simulink model "sm_scissor_lift_testenv"  (R2021a)
settings: Solver=ode15s  StartTime=0.0  StopTime=50  FixedStep=5e-3  MaxStep=1e-2  RelTol=1e-3  AbsTol=1e-4  EnableMultiTasking=on
PreLoadFcn:
  | if(~exist('SCL_Par'))
  |   SCL_Par = sm_scissor_lift_param;
  | end
PostLoadFcn:
  | warning('off','mech2:compiler:topologyAnalysis:DanglingBlock');
  | warning('off','sm:sli:setup:compile:LocalSolverNotSupported');
  | warning('off','MATLAB:subscripting:noSubscriptsSpecified');
StartFcn:
  | tic;
StopFcn:
  | Elapsed_Sim_Time = toc;
  | %disp(['Elapsed Sim Time = ' num2str(Elapsed_Sim_Time')]);
values from neighbouring files (symbols this model uses):
  lift_extra_mass = 0    [startup_sm_scissor_lift.m]
undefined symbols (not defined in the file or in its folder): Local, sigbuilder_block, X, Y, Z
libraries: sm_lib x116, sm_scissor_lift_lib x29, nesl_utility x26, fl_lib x8, sh_lib x4, Contact_Forces_Lib x4, simulink x1
(part 1 of 6)
CloseFcn:
  | try,close(h1_sm_scissor_lift_testenv),end
  | clear h1_Scissor_Lift
  | try,close(h2_sm_scissor_lift_testenv),end
  | clear h2_Scissor_Lift
  | try,close(hUI_sm_scissor_lift_testenv),end
  | clear hUI_sm_scissor_lift_testenv
  | 
  | clear simlog_sm_scissor_lift_testenv
  | clear logsout_sm_scissor_lift_testenv
Description:
  | Scissor Lift Test Environment
  | 
  | Copyright 2014-2021 The MathWorks, Inc.
settings Model: Creator=smiller  LastModifiedBy=smiller
settings SolverCC: AutoScaleAbsTol=off  ConcurrentTasks=on  AlgebraicLoopSolver=TrustRegion  AutoInsertRateTranBlk=on  InsertRTBMode=Never (minimum delay)
settings DataIOCC: MaxDataPoints=10000  SaveFormat=StructureWithTime  ReturnWorkspaceOutputs=off  SignalLoggingName=logsout_sm_scissor_lift_testenv
settings OptimizationCC: BlockReduction=off  OptimizeBlockIOStorage=off  BufferReuse=off  GlobalBufferReuse=off  ExpressionFolding=off  ExpressionDepthLimit=2147483647  LocalBlockOutputs=off  OptimizeDataStoreBuffers=off  BusAssignmentInplaceUpdate=off
settings DebuggingCC: AlgebraicLoopMsg=error  UnderspecifiedInitializationDetection=Classic  MergeDetectMultiDrivingBlocksExec=none  SolverPrmCheckMsg=warning  AllowSymbolicDim=off  StateNameClashWarn=warning  PregeneratedLibrarySubsystemCodeDiagnostic=none  SFUnexpectedBacktrackingDiag=warning  SFNoUnconditionalDefaultTransitionDiag=warning  SFExecutionAtInitializationDiag=none  SFMachineParentedDataDiag=warning  ArithmeticOperatorsInVariantConditions=warning
settings ModelReferenceCC: PropagateSignalLabelsOutOfModel=off
settings SFSimCC: SimUseLocalCustomCode=off  CustomCodeUndefinedFunction=UseInterfaceOnly
settings RTWCC: Description=Generic Real-Time Target  RTWUseLocalCustomCode=off  RTWCompilerOptimization=on
settings CodeAppCC: StateflowObjectComments=on
settings GRTTargetCC: TargetLangStandard=C89/C90 (ANSI)
settings ConfigComp: CovMetricSettings=dw  CovSaveCumulativeToWorkspaceVar=on  CovSaveSingleToWorkspaceVar=on  CovExternalEMLEnable=off  CovSFcnEnable=off
settings SimscapeCC: SimscapeNormalizeSystem=off  SimscapeLogType=all  SimscapeLogSimulationStatistics=on  SimscapeLogName=simlog_sm_scissor_lift_testenv  SimscapeLogDataHistory=10000
settings ConfigurationSet: Description=SimMechanics 2G
settings DiagnosticsConfigSet: SimMechanicsUnconnectedFramePorts=none  SimMechanicsRigidlyBoundBlock=none
settings ExplorerConfigSet: InternalSimMechanicsExplorerSettings="<ExplorerConfiguration><canonicalview>default</canonicalview><AnimationSetting><BasePlaybackSpeed>1.0</BasePlaybackSpeed><PlaybackSpeedFactor>4.0</PlaybackSpeedFactor></AnimationSetting><TilePanel><TileInfo><Tiles Columns=\"2\" Count=\"3\" Rows=\"2\"><Column Left=\"2\" Weight=\"0.5\"/><Column Left=\"319\" Weight=\"0.5\"/><Column Left=\"636\"/><Row Top=\"2\" Weight=\"0.434\"/><Row Top=\"317\" Weight=\"0.566\"/><Row Top=\"726\"/><Tile Height=\"1\" Width=\"2\" X=\"0\" Y=\"0\"/><Tile Height=\"1\" Width=\"1\" X=\"0\" Y=\"1\"/><Tile Height=\"1\" Width=\"1\" X=\"1\" Y=\"1\"/></Tiles></TileInfo><SceneInfo><SceneViewer><BGColor><R>1</R><G>1</G><B>1</B></BGColor><Camera><DoPerspective>on</DoPerspective><Position><X>0.78465604483800933</X><Y>0.74998508124070185</Y><Z>5.7969918564344418</Z></Position><Center><X>1.7378942726283986</X><Y>1.0522050029517593</Y><Z>5.7969918564344409</Z></Center><Up><X>4.5985052243862679e-16</X><Y>5.259771773997932e-16</Y><Z>1</Z></Up><ViewLimDist>1</ViewLimDist><YLim>0.46630765815499858</YLim><XLim>0.95242577237540549</XLim></Camera></SceneViewer><SceneViewer><BGColor><R>1</R><G>1</G><B>1</B></BGColor><Camera><DoPerspective>off</DoPerspective><Position><X>0.019999865036961495</X><Y>-3.7807005970336149e-08</Y><Z>11.13211424643969</Z></Position><Center><X>0.019999865036961495</X><Y>-3.7807005970336149e-08</Y><Z>3.4806946063285658</Z></Center><Up><X>0</X><Y>1</Y><Z>-0</Z></Up><ViewLimDist>1</ViewLimDist><YLim>6.1531750545026354</YLim><XLim>4.7379447919670294</XLim></Camera></SceneViewer><SceneViewer><BGColor><R>1</R><G>1</G><B>1</B></BGColor><Camera><DoPerspective>off</DoPerspective><Position><X>1.0546030947508469</X><Y>-9.8853504412716475</Y><Z>4.0090833581699536</Z></Position><Center><X>1.0546030947508469</X><Y>-2.1392246596363407e-07</Y><Z>4.0090833581699536</Z></Center><Up><X>0</X><Y>-0</Y><Z>1</Z></Up><ViewLimDist>1</ViewLimDist><YLim>4.9840717941471349</YLim><XLim>3.8377352814932939</XLim></Camera></SceneViewer></SceneInfo></TilePanel><MechEditorPanel><Cameras><Camera><Id>Camera1</Id><Value><Name>Platform</Name><NativeCamera><PositionTrackingFeature>Scissor_Lift.Platform.Fixed.Cage.Transform_Camera.F</PositionTrackingFeature><CenterTrackingFeature>Scissor_Lift.Platform.Fixed.Cage.Transform_Camera.F</CenterTrackingFeature><UpVectorTrackingFeature>Scissor_Lift.Platform.Fixed.Cage.Transform_Camera.F</UpVectorTrackingFeature><CenterTrackingOrigin>off</CenterTrackingOrigin><CenterTrackingDirection>-Y</CenterTrackingDirection><UpVectorTrackingDirection>+Z</UpVectorTrackingDirection></NativeCamera></Value></Camera></Cameras><GfxPanelCameraMap><MapElement CameraMLId=\"Camera1\" GfxPanelIndex=\"0\"/></GfxPanelCameraMap><VideoCreator><PlaybackSpeedRatio>1.0</PlaybackSpeedRatio><FrameRate>30</FrameRate><VideoFormat>Motion JPEG AVI</VideoFormat><FrameSize>auto</FrameSize></VideoCreator></MechEditorPanel></ExplorerConfiguration>"

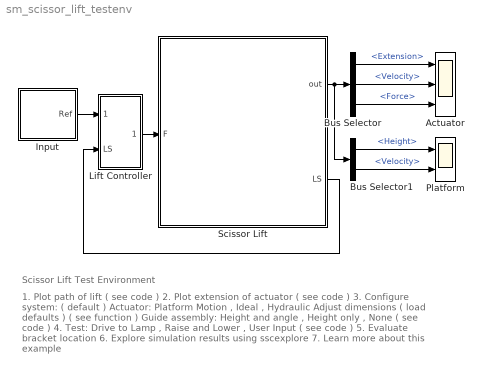
== system sm_scissor_lift_testenv ==
  note: Scissor Lift Test Environment
  note: 1. Plot path of lift ( see code )
      | 2. Plot extension of actuator ( see code )
      | 3. Configure system: ( default )
      | Actuator: Platform Motion , Ideal , Hydraulic
      | Adjust dimensions ( load defaults ) ( see function )
      | Guide assembly: Height and angle , Height only , None ( see code )
      | 4. Test: Drive to Lamp , Raise and Lower , User Input ( see code )
      | 5. Evaluate bracket location
      | 6. Explore simulation results using sscexplore
      | 7. Learn more about this example
  Actuator : Scope  NumInputPorts=3
  Bus Selector : BusSelector  OutputSignals=Actuator.Extension,Actuator.Velocity,Actuator.Force
  Bus Selector1 : BusSelector  OutputSignals=Platform.Height,Platform.Velocity
  Input : Subsystem  Variant=on  VariantControlMode=label  VariantControl=Variant1  LabelModeActiveChoice=Test_Input
      settings: AttributesFormatString=%<ActiveVariant>
      mask Display:
      | blk = find_system(gcbh, 'SearchDepth', 1, 'Parent', gcb, 'VariantObject', get_param(gcb,'activevariant'));
      | eval(get_param(blk, 'MaskDisplay'));
  Lift Controller : Subsystem
  Platform : Scope  NumInputPorts=2
  Scissor Lift : Subsystem  Tag=PublishSubsystem
      mask Display:
      | image('Scissor_Lift_3Stage_Full_IMAGE.jpg');
      | %port_label('input',1,'F');
      | %port_label('output',1,'pv');
  wires:
  Lift Controller/1(Cmd) -> Scissor Lift/1(F)
  Bus Selector/2 -> Actuator/2  "<Velocity>"
  Scissor Lift/2(LS) -> Lift Controller/2(LS)
  Input/1(" Ref") -> Lift Controller/1(Ref)
  Bus Selector/3 -> Actuator/3  "<Force>"
  Scissor Lift/1(out) -> Bus Selector1/1, Bus Selector/1
  Bus Selector1/1 -> Platform/1  "<Height>"
  Bus Selector1/2 -> Platform/2  "<Velocity>"
  Bus Selector/1 -> Actuator/1  "<Extension>"

== system sm_scissor_lift_testenv/Input ==
  Dashboard : Subsystem  VariantControl=Dashboard
      mask Display: image(imread('Scissor_Lift_Input_Dashboard_IMAGE.jpg'));
  Input : Subsystem  VariantControl=Test_Input
      mask Display: image('Scissor_Lift_Input_TestSequence_IMAGE.jpg');
  " Ref" : Outport  VectorParamsAs1DForOutWhenUnconnected=off

== system sm_scissor_lift_testenv/Lift Controller ==
  note: Copyright 2011-2021 The MathWorks, Inc.
  Ref : Inport
  LS : Inport  Port=2
  Bus Creator : BusCreator  Inputs=4
  Bus Selector : BusSelector  OutputSignals=Lift,Drive,Steer,Extend
  Bus Selector1 : BusSelector  OutputSignals=LS Height
  Full : Constant  Value=10
  Gain : Gain  Gain=0.5
  Gain1 : Gain  Gain=0.5
  Integrator : Integrator
  Integrator1 : Integrator
  Limit : Constant  Value=5
  Max Trq : Switch  Criteria=u2 > Threshold
  Product : Product
  Saturation : Saturate  UpperLimit=SCL_Par.Platform.Ext.Length*0.6/100  LowerLimit=0
  Cmd : Outport  VectorParamsAs1DForOutWhenUnconnected=off
  wires:
  Ref/1 -> Bus Selector/1
  LS/1 -> Bus Selector1/1
  Bus Selector/1 -> Bus Creator/1  "<Lift>"
  Bus Selector/2 -> Product/2  "<Drive>"
  Bus Selector/3 -> Gain/1  "<Steer>"
  Bus Creator/1 -> Cmd/1  "Cmd"
  Full/1 -> Max Trq/3
  Limit/1 -> Max Trq/1
  Max Trq/1 -> Product/1
  Product/1 -> Bus Creator/2  "Drive"
  Bus Selector1/1 -> Max Trq/2  "<LS Height>"
  Gain/1 -> Integrator/1
  Integrator/1 -> Bus Creator/3  "Steer"
  Bus Selector/4 -> Gain1/1  "<Extend>"
  Gain1/1 -> Integrator1/1
  Integrator1/1 -> Saturation/1
  Saturation/1 -> Bus Creator/4  "Extend"

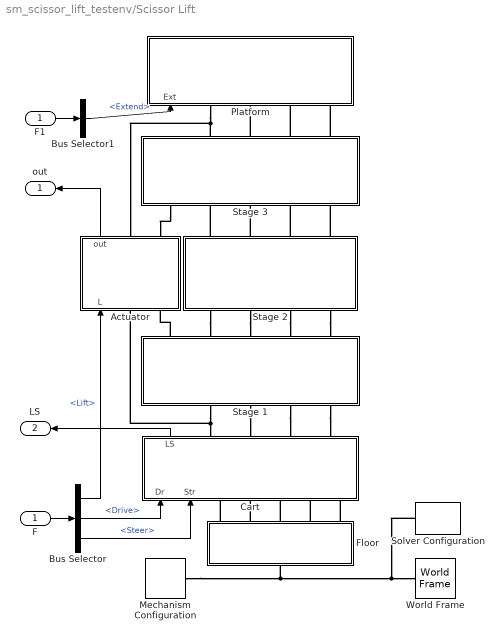
== system sm_scissor_lift_testenv/Scissor Lift ==
  F : Inport
  Actuator : Subsystem
      mask Display:
      | curblk = gcb;
      | blk = find_system([curblk '/Actuator'], 'SearchDepth', 1, 'Parent', [curblk '/Actuator'], 'VariantObject', get_param([curblk '/Actuator'],'activevariant'));
      | eval(char(get_param(blk, 'MaskDisplay')));
  Bus Selector : BusSelector  OutputSignals=Lift,Drive,Steer
  Bus Selector1 : BusSelector  OutputSignals=Extend
  Cart : Subsystem
      mask Display: image('sm_scissor_lift_cart_IMAGE.png');
  F1 : InportShadow
  Floor : Subsystem  Tag=PublishSubsystem
      mask Display: image('sm_scissor_lift_floor_IMAGE.png');
  Mechanism Configuration : sm_lib/Utilities/Mechanism Configuration  UniformGravity=Constant  GravityVector=[0 0 -9.81]  GravityVectorUnits=m/s^2  GravityUnits=m/s^2  LinearizationDelta=0.001  JointModeTransitionNonlinearIterations=2
  Platform : Subsystem
      mask Display: image('sm_scissor_lift_platform_IMAGE.png');
  Solver Configuration : nesl_utility/Solver Configuration  PhysicalDomain=network_engine_domain  SubClassName=solver  LeftPortType=input  RightPortType=generic  Tones=[]  Harmonics=[]  SimulateNoise=off  Profile=off  UseLocalSampling=off  EnableSwitchedLinearOptims=on  FrequencyDomain=off  UseCCode=off  RelTol=0.001  AbsTol=1e-06  MinStep=1e-09  ToWorkspace=off  RevertToSquareIcSolve=off  NumHomotopyIterations=100  PhasorMode=off  PhasorModeNumHarmonics=1  DoDC=off  ResidualTolerance=1e-9  UseLocalSolver=off  LocalSolverChoice=NE_BACKWARD_EULER_ADVANCER  LocalSolverSampleTime=.001  DoFixedCost=off  MaxNonlinIter=3  MaxModeIter=2  ComputeImpulses=off  ImpulseIterations=2  LinearAlgebra=Sparse  EquationFormulation=NE_TIME_EF  DelaysMemoryBudget=1024  AutomaticFiltering=on  FilteringTimeConstant=0.001  PartitionStorageMethod=AS_NEEDED  PartitionMemoryBudget=1024  PartitionMethod=FAST
      settings: SourceProductBaseCode=PW,SS
  Stage 1 : Subsystem  Tag=PublishSubsystem
      mask Display: image('sm_scissor_lift_stage1_IMAGE.png');
  Stage 2 : Subsystem
      mask Display: image('sm_scissor_lift_stage2_IMAGE.png');
  Stage 3 : Subsystem
      mask Display: image('sm_scissor_lift_stage3_IMAGE.png');
  World Frame : sm_lib/Frames and Transforms/World Frame
  out : Outport  VectorParamsAs1DForOutWhenUnconnected=off
  LS : Outport  Port=2  VectorParamsAs1DForOutWhenUnconnected=off
  wires:
  Actuator/1(out) -> out/1
  F/1 -> Bus Selector/1
  Bus Selector/1 -> Actuator/1(L)  "<Lift>"
  Bus Selector/2 -> Cart/1(Dr)  "<Drive>"
  Bus Selector/3 -> Cart/2(Str)  "<Steer>"
  Cart/1(LS) -> LS/1
  F1/1 -> Bus Selector1/1
  Bus Selector1/1 -> Platform/1(Ext)  "<Extend>"
  connections:
  Stage 1/LConn1 -- Actuator/LConn2
  Stage 3/RConn1 -- Actuator/RConn2
  Actuator/LConn1 -- Stage 1/RConn2 -- Cart/RConn1
  Stage 1/RConn3 -- Cart/RConn2
  Stage 1/RConn4 -- Cart/RConn3
  Stage 1/RConn5 -- Cart/RConn4
  Mechanism Configuration/RConn1 -- Solver Configuration/RConn1 -- World Frame/RConn1 -- Floor/RConn1
  Platform/LConn1 -- Stage 3/LConn2 -- Actuator/RConn1
  Stage 3/LConn3 -- Platform/LConn2
  Stage 3/LConn4 -- Platform/LConn3
  Stage 3/LConn5 -- Platform/LConn4
  Floor/LConn4 -- Cart/LConn4
  Floor/LConn3 -- Cart/LConn3
  Floor/LConn1 -- Cart/LConn1
  Floor/LConn2 -- Cart/LConn2
  Floor/LConn5 -- Cart/LConn5
  Stage 2/LConn4 -- Stage 3/RConn5
  Stage 2/LConn2 -- Stage 3/RConn3
  Stage 2/RConn1 -- Stage 1/LConn2
  Stage 2/RConn2 -- Stage 1/LConn3
  Stage 2/LConn1 -- Stage 3/RConn2
  Stage 2/RConn3 -- Stage 1/LConn4
  Stage 2/RConn4 -- Stage 1/LConn5
  Stage 2/LConn3 -- Stage 3/RConn4

== system sm_scissor_lift_testenv/Input/Dashboard ==
  note: Use Simulation Pacing to make the simulation in soft real-time so that you can use the manual controls below
  Bus Creator : BusCreator  Inputs=4
  Drive : Constant  Value=0
  Extend : Constant  Value=0
  Lift : Constant  Value=0
  Push Button : PushButtonBlock  ButtonText=Up
  Push Button1 : PushButtonBlock  ButtonText=Down  OnValue=-1
  Push Button2 : PushButtonBlock  ButtonText=Forward
  Push Button3 : PushButtonBlock  ButtonText=Reverse  OnValue=-1
  Push Button4 : PushButtonBlock  ButtonText=Left
  Push Button5 : PushButtonBlock  ButtonText=Right  OnValue=-1
  Push Button6 : PushButtonBlock  ButtonText=Retract  OnValue=-1
  Push Button7 : PushButtonBlock  ButtonText=Extend
  Steer : Constant  Value=0
  Ref : Outport  VectorParamsAs1DForOutWhenUnconnected=off
  wires:
  Lift/1 -> Bus Creator/1  "Lift"
  Drive/1 -> Bus Creator/2  "Drive"
  Bus Creator/1 -> Ref/1  "Ref"
  Steer/1 -> Bus Creator/3  "Steer"
  Extend/1 -> Bus Creator/4  "Extend"

== system sm_scissor_lift_testenv/Input/Input ==
  Bus Creator : BusCreator  Inputs=4
  Signal Builder : Subsystem  Tag=STV Subsys  LoadFcn=sigbuilder_block('load');  StartFcn=sigbuilder_block('start');  StopFcn=sigbuilder_block('stop');  ClipboardFcn=sigbuilder_block('clipboard');  mask(Sigbuilder block){tuvar=[0:10]}
      mask help: Simulink:masks:SigbuilderBlock_MD
      mask init:
      | if ~strcmp(get_param(bdroot(gcbh),'SimulationStatus'),'stopped') tuvar = sigbuilder_block('maskInit'); end
      settings: CopyFcn=sigbuilder_block('copy');  DeleteFcn=sigbuilder_block('delete');  ModelCloseFcn=sigbuilder_block('modelClose');  PreSaveFcn=sigbuilder_block('preSave');  PauseFcn=sigbuilder_block('pause');  ContinueFcn=sigbuilder_block('continue');  NameChangeFcn=sigbuilder_block('namechange');  OpenFcn=sigbuilder_block('open',[49.8 117.6 550.8 438.6 ]);  CloseFcn=sigbuilder_block('close');
      mask Display: plot(0, 0, 100, 100,[2, 2, 32, 32, 2], [68, 8, 8, 68, 68],[32, 2], [38, 38], [32, 19, 2],[53, 60, 44], [32, 17, 17, 2],[16, 16, 31, 31]);txt = getActiveGroup(gcbh);text(2, 100, txt,'verticalAlignment', 'top');
  Ref : Outport  VectorParamsAs1DForOutWhenUnconnected=off
  wires:
  Signal Builder/3(Steer) -> Bus Creator/3  "Steer"
  Bus Creator/1 -> Ref/1  "Ref"
  Signal Builder/2(Drive) -> Bus Creator/2  "Drive"
  Signal Builder/1(Lift) -> Bus Creator/1  "Lift"
  Signal Builder/4(Extend) -> Bus Creator/4  "Extend"

== system sm_scissor_lift_testenv/Scissor Lift/Actuator ==
  L : Inport
  Actuator : Subsystem  Variant=on  VariantControlMode=label  LabelModeActiveChoice=Ideal
      settings: AttributesFormatString=%<ActiveVariant>
      mask Display:
      | curblk = gcb;
      | 
      | parentblk = get_param(curblk,'Parent');
      | parblk_name = char(get_param(parentblk,'Name'));
      | set_param(parentblk,'Name',parblk_name);
      | 
      | 
      | blk = find_system(gcbh, 'SearchDepth', 1, 'Parent', gcb, 'VariantObject', get_param(gcb,'activevariant'));
      | eval(get_param(blk, 'MaskDisplay'));
  Cylinder Collar : sm_scissor_lift_lib/Collar  collar_length=SCL_Par.Act.Collar.Length  collar_radius=SCL_Par.Act.Collar.Radius  cylinder_length=SCL_Par.Act.Cylinder.Length  cylinder_radius=SCL_Par.Act.Cylinder.Radius  cylinder_ori=Local +Z  material_density=SCL_Par.Act.Collar.Density  material_color=SCL_Par.Act.Collar.Color  material_opacity=SCL_Par.Act.Collar.Opacity
      settings: SourceProductName=Simscape Scissor Lift Library
  Piston : Subsystem
      mask Display: image('Piston_Shaft_IMAGE.jpg');
  Piston Collar : sm_scissor_lift_lib/Collar  collar_length=SCL_Par.Act.Collar.Length  collar_radius=SCL_Par.Act.Collar.Radius  cylinder_length=SCL_Par.Act.Piston_Seat.Length  cylinder_radius=SCL_Par.Act.Piston_Seat.Radius  cylinder_ori=Local -Z  material_density=SCL_Par.Act.Collar.Density  material_color=SCL_Par.Act.Collar.Color  material_opacity=SCL_Par.Act.Collar.Opacity
      settings: SourceProductName=Simscape Scissor Lift Library
  Rev Bracket1 Cyl : sm_lib/Joints/Revolute Joint  JointMode=Normal  SenseConstraintForce=off  SenseConstraintForceX=off  SenseConstraintForceY=off  SenseConstraintForceZ=off  SenseConstraintTorque=off  SenseConstraintTorqueX=off  SenseConstraintTorqueY=off  SenseConstraintTorqueZ=off  SenseTotalForce=off  SenseTotalForceX=off  SenseTotalForceY=off  SenseTotalForceZ=off  SenseTotalTorque=off  SenseTotalTorqueX=off  SenseTotalTorqueY=off  SenseTotalTorqueZ=off  CompositeWrenchDir=FollowerOnBase  CompositeWrenchFrame=BaseFrame  EquilibriumPosition=0  EquilibriumPositionUnits=rad  SpringStiffness=0  SpringStiffnessUnits=N*m/rad  DampingCoefficient=0  DampingCoefficientUnits=N*m/(rad/s)  TorqueActuationMode=NoTorque  MotionActuationMode=ComputedMotion  SensePosition=off  SenseVelocity=off  SenseAcceleration=off  SenseTorqueForce=off  SenseLowerLimitTorqueForce=off  SenseUpperLimitTorqueForce=off  LowerLimitSpecify=off  LowerLimitBound=-90  LowerLimitBoundUnits=deg  LowerLimitStiffness=1e4  LowerLimitStiffnessUnits=N*m/deg  LowerLimitDamping=10  LowerLimitDampingUnits=N*m/(deg/s)  LowerLimitTransitionRegionWidth=0.1  LowerLimitTransitionRegionWidthUnits=deg  UpperLimitSpecify=off  UpperLimitBound=90  UpperLimitBoundUnits=deg  UpperLimitStiffness=1e4  UpperLimitStiffnessUnits=N*m/deg  UpperLimitDamping=10  UpperLimitDampingUnits=N*m/(deg/s)  UpperLimitTransitionRegionWidth=0.1  UpperLimitTransitionRegionWidthUnits=deg  PositionTargetSpecify=off  PositionTargetPriority=High  PositionTargetValue=0  PositionTargetValueUnits=rad  VelocityTargetSpecify=off  VelocityTargetPriority=High  VelocityTargetValue=0  VelocityTargetValueUnits=rad/s
  Rev Bracket2 Cyl : sm_lib/Joints/Revolute Joint  JointMode=Normal  SenseConstraintForce=off  SenseConstraintForceX=off  SenseConstraintForceY=off  SenseConstraintForceZ=off  SenseConstraintTorque=off  SenseConstraintTorqueX=off  SenseConstraintTorqueY=off  SenseConstraintTorqueZ=off  SenseTotalForce=off  SenseTotalForceX=off  SenseTotalForceY=off  SenseTotalForceZ=off  SenseTotalTorque=off  SenseTotalTorqueX=off  SenseTotalTorqueY=off  SenseTotalTorqueZ=off  CompositeWrenchDir=FollowerOnBase  CompositeWrenchFrame=BaseFrame  EquilibriumPosition=0  EquilibriumPositionUnits=rad  SpringStiffness=0  SpringStiffnessUnits=N*m/rad  DampingCoefficient=0  DampingCoefficientUnits=N*m/(rad/s)  TorqueActuationMode=NoTorque  MotionActuationMode=ComputedMotion  SensePosition=off  SenseVelocity=off  SenseAcceleration=off  SenseTorqueForce=off  SenseLowerLimitTorqueForce=off  SenseUpperLimitTorqueForce=off  LowerLimitSpecify=off  LowerLimitBound=-90  LowerLimitBoundUnits=deg  LowerLimitStiffness=1e4  LowerLimitStiffnessUnits=N*m/deg  LowerLimitDamping=10  LowerLimitDampingUnits=N*m/(deg/s)  LowerLimitTransitionRegionWidth=0.1  LowerLimitTransitionRegionWidthUnits=deg  UpperLimitSpecify=off  UpperLimitBound=90  UpperLimitBoundUnits=deg  UpperLimitStiffness=1e4  UpperLimitStiffnessUnits=N*m/deg  UpperLimitDamping=10  UpperLimitDampingUnits=N*m/(deg/s)  UpperLimitTransitionRegionWidth=0.1  UpperLimitTransitionRegionWidthUnits=deg  PositionTargetSpecify=off  PositionTargetPriority=High  PositionTargetValue=0  PositionTargetValueUnits=rad  VelocityTargetSpecify=off  VelocityTargetPriority=High  VelocityTargetValue=0  VelocityTargetValueUnits=rad/s
  Transform From Cart : sm_lib/Frames and Transforms/Rigid Transform  TranslationMethod=None  TranslationStandardOffset=0  TranslationLengthUnit=m  TranslationStandardAxis=+X  TranslationCartesianOffset=[0 0 0]  TranslationROffset=0  TranslationROffsetUnits=m  TranslationZOffset=0  TranslationZOffsetUnits=m  TranslationThetaOffset=0  TranslationThetaOffsetUnits=deg  RotationMethod=StandardAxis  RotationAngleUnits=deg  RotationStandardAxis=+X  RotationAngle=90  RotationArbitraryAxis=[0 0 1]  FollAlignAxisA=+X  BaseAlignAxisA=+Y  FollAlignAxisB=+Y  BaseAlignAxisB=+Z  RotationSequenceAxes=FollowerAxes  RotationSequence=XYX  RotationSequenceAngles=[0 0 0]  RotationSequenceAnglesUnits=deg  RotationMatrix=[1 0 0; 0 1 0; 0 0 1]
  Transform From Platform : sm_lib/Frames and Transforms/Rigid Transform  TranslationMethod=None  TranslationStandardOffset=0  TranslationLengthUnit=m  TranslationStandardAxis=+X  TranslationCartesianOffset=[0 0 0]  TranslationROffset=0  TranslationROffsetUnits=m  TranslationZOffset=0  TranslationZOffsetUnits=m  TranslationThetaOffset=0  TranslationThetaOffsetUnits=deg  RotationMethod=StandardAxis  RotationAngleUnits=deg  RotationStandardAxis=+X  RotationAngle=90  RotationArbitraryAxis=[0 0 1]  FollAlignAxisA=+X  BaseAlignAxisA=+Y  FollAlignAxisB=+Y  BaseAlignAxisB=+Z  RotationSequenceAxes=FollowerAxes  RotationSequence=XYX  RotationSequenceAngles=[0 0 0]  RotationSequenceAnglesUnits=deg  RotationMatrix=[1 0 0; 0 1 0; 0 0 1]
  C : PMIOPort  Side=Left
  P : PMIOPort  Port=2  Side=Right
  F : PMIOPort  Port=3  Side=Right
  B : PMIOPort  Port=4  Side=Left
  out : Outport  VectorParamsAs1DForOutWhenUnconnected=off
  wires:
  L/1 -> Actuator/1(L)
  Actuator/1(Out) -> out/1
  connections:
  Cylinder Collar/LConn1 -- Rev Bracket1 Cyl/RConn1
  Piston Collar/RConn1 -- Piston/LConn1
  Rev Bracket2 Cyl/RConn1 -- Piston Collar/LConn1
  F/RConn1 -- Rev Bracket2 Cyl/LConn1
  Rev Bracket1 Cyl/LConn1 -- B/RConn1
  Actuator/RConn2 -- Piston/RConn1
  Actuator/LConn2 -- Cylinder Collar/RConn1
  C/RConn1 -- Transform From Cart/LConn1
  P/RConn1 -- Transform From Platform/LConn1
  Transform From Cart/RConn1 -- Actuator/LConn1
  Transform From Platform/RConn1 -- Actuator/RConn1

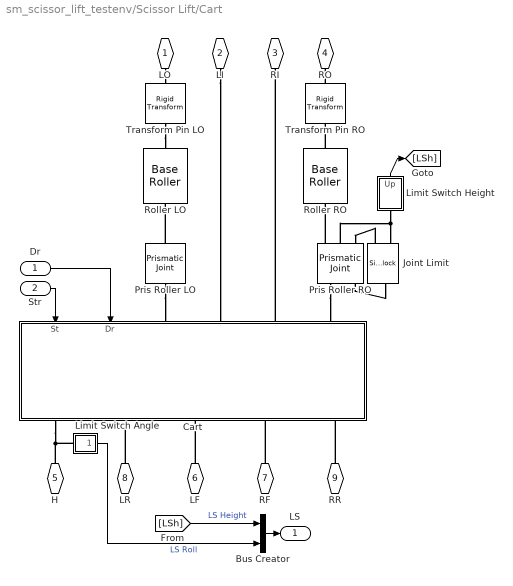
== system sm_scissor_lift_testenv/Scissor Lift/Cart ==
  Dr : Inport
  Str : Inport  Port=2
  Bus Creator : BusCreator  Inputs=2
  Cart : Subsystem
      mask Display: image('Scissor_Lift_Cart_IMAGE.jpg');
  Joint Limit : SimscapeComponentBlock  SourceFile=translational_hardstop  ComponentPath=translational_hardstop  ComponentVariants=translational_hardstop  ComponentVariantNames=translational_hardstop  ClassName=translational_hardstop  SchemaVersion=1  upper_bnd=SCL_Par.Roller.Hardstop.UB cm  lower_bnd=SCL_Par.Roller.Hardstop.LB cm  stiff_up=SCL_Par.Roller.Hardstop.Stiffness N/m  stiff_low=SCL_Par.Roller.Hardstop.Stiffness N/m  D_up=SCL_Par.Roller.Hardstop.Damping N/(m/s)  D_low=SCL_Par.Roller.Hardstop.Damping N/(m/s)
      settings: CopyFcn=simscape.engine.sli.internal.componentblockcallback(gcbh,'COPY')  PreCopyFcn=simscape.engine.sli.internal.componentblockcallback(gcbh,'PRECOPY')  PreDeleteFcn=simscape.engine.sli.internal.componentblockcallback(gcbh,'PREDELETE')
      mask Type: Translational Hard Stop
  Limit Switch Angle : Subsystem
  Limit Switch Height : Subsystem
  Pris Roller LO : sm_lib/Joints/Prismatic Joint  JointMode=Normal  SenseConstraintForce=off  SenseConstraintForceX=off  SenseConstraintForceY=off  SenseConstraintForceZ=off  SenseConstraintTorque=off  SenseConstraintTorqueX=off  SenseConstraintTorqueY=off  SenseConstraintTorqueZ=off  SenseTotalForce=off  SenseTotalForceX=off  SenseTotalForceY=off  SenseTotalForceZ=off  SenseTotalTorque=off  SenseTotalTorqueX=off  SenseTotalTorqueY=off  SenseTotalTorqueZ=off  CompositeWrenchDir=FollowerOnBase  CompositeWrenchFrame=BaseFrame  EquilibriumPosition=0  EquilibriumPositionUnits=m  SpringStiffness=0  SpringStiffnessUnits=N/m  DampingCoefficient=0  DampingCoefficientUnits=N/(m/s)  TorqueActuationMode=NoTorque  MotionActuationMode=ComputedMotion  SensePosition=off  SenseVelocity=off  SenseAcceleration=off  SenseTorqueForce=off  SenseLowerLimitTorqueForce=off  SenseUpperLimitTorqueForce=off  LowerLimitSpecify=off  LowerLimitBound=-1  LowerLimitBoundUnits=m  LowerLimitStiffness=1e6  LowerLimitStiffnessUnits=N/m  LowerLimitDamping=1e3  LowerLimitDampingUnits=N/(m/s)  LowerLimitTransitionRegionWidth=1e-4  LowerLimitTransitionRegionWidthUnits=m  UpperLimitSpecify=off  UpperLimitBound=1  UpperLimitBoundUnits=m  UpperLimitStiffness=1e6  UpperLimitStiffnessUnits=N/m  UpperLimitDamping=1e3  UpperLimitDampingUnits=N/(m/s)  UpperLimitTransitionRegionWidth=1e-4  UpperLimitTransitionRegionWidthUnits=m  PositionTargetSpecify=off  PositionTargetPriority=High  PositionTargetValue=SCL_Par.Init.Roller_Position  PositionTargetValueUnits=cm  VelocityTargetSpecify=off  VelocityTargetPriority=High  VelocityTargetValue=0  VelocityTargetValueUnits=m/s
  Pris Roller RO : sm_lib/Joints/Prismatic Joint  JointMode=Normal  SenseConstraintForce=off  SenseConstraintForceX=off  SenseConstraintForceY=off  SenseConstraintForceZ=off  SenseConstraintTorque=off  SenseConstraintTorqueX=off  SenseConstraintTorqueY=off  SenseConstraintTorqueZ=off  SenseTotalForce=off  SenseTotalForceX=off  SenseTotalForceY=off  SenseTotalForceZ=off  SenseTotalTorque=off  SenseTotalTorqueX=off  SenseTotalTorqueY=off  SenseTotalTorqueZ=off  CompositeWrenchDir=FollowerOnBase  CompositeWrenchFrame=BaseFrame  EquilibriumPosition=0  EquilibriumPositionUnits=m  SpringStiffness=0  SpringStiffnessUnits=N/m  DampingCoefficient=0  DampingCoefficientUnits=N/(m/s)  TorqueActuationMode=InputTorque  MotionActuationMode=ComputedMotion  SensePosition=on  SenseVelocity=on  SenseAcceleration=off  SenseTorqueForce=off  SenseLowerLimitTorqueForce=off  SenseUpperLimitTorqueForce=off  LowerLimitSpecify=off  LowerLimitBound=-1  LowerLimitBoundUnits=m  LowerLimitStiffness=1e6  LowerLimitStiffnessUnits=N/m  LowerLimitDamping=1e3  LowerLimitDampingUnits=N/(m/s)  LowerLimitTransitionRegionWidth=1e-4  LowerLimitTransitionRegionWidthUnits=m  UpperLimitSpecify=off  UpperLimitBound=1  UpperLimitBoundUnits=m  UpperLimitStiffness=1e6  UpperLimitStiffnessUnits=N/m  UpperLimitDamping=1e3  UpperLimitDampingUnits=N/(m/s)  UpperLimitTransitionRegionWidth=1e-4  UpperLimitTransitionRegionWidthUnits=m  PositionTargetSpecify=off  PositionTargetPriority=High  PositionTargetValue=0  PositionTargetValueUnits=m  VelocityTargetSpecify=off  VelocityTargetPriority=High  VelocityTargetValue=0  VelocityTargetValueUnits=m/s
  Roller LO : sm_scissor_lift_lib/Base Roller  roller_length=SCL_Par.Roller.Roller_Length  roller_radius=SCL_Par.Roller.Roller_Radius  shaft_length=SCL_Par.Roller.Shaft_Length  shaft_radius=SCL_Par.Roller.Shaft_Radius  material_density=SCL_Par.Roller.Density  material_color=SCL_Par.Roller.Color  material_opacity=SCL_Par.Roller.Opacity
      settings: SourceProductName=Simscape Scissor Lift Library
  Roller RO : sm_scissor_lift_lib/Base Roller  roller_length=SCL_Par.Roller.Roller_Length  roller_radius=SCL_Par.Roller.Roller_Radius  shaft_length=SCL_Par.Roller.Shaft_Length  shaft_radius=SCL_Par.Roller.Shaft_Radius  material_density=SCL_Par.Roller.Density  material_color=SCL_Par.Roller.Color  material_opacity=SCL_Par.Roller.Opacity
      settings: SourceProductName=Simscape Scissor Lift Library
  Transform Pin LO : sm_lib/Frames and Transforms/Rigid Transform  TranslationMethod=None  TranslationStandardOffset=0  TranslationLengthUnit=m  TranslationStandardAxis=+Z  TranslationCartesianOffset=[0 0 0]  TranslationROffset=0  TranslationROffsetUnits=m  TranslationZOffset=0  TranslationZOffsetUnits=m  TranslationThetaOffset=0  TranslationThetaOffsetUnits=deg  RotationMethod=StandardAxis  RotationAngleUnits=deg  RotationStandardAxis=+Z  RotationAngle=180  RotationArbitraryAxis=[0 0 1]  FollAlignAxisA=+X  BaseAlignAxisA=+Y  FollAlignAxisB=+Y  BaseAlignAxisB=+Z  RotationSequenceAxes=FollowerAxes  RotationSequence=XYX  RotationSequenceAngles=[0 0 0]  RotationSequenceAnglesUnits=deg  RotationMatrix=[1 0 0; 0 1 0; 0 0 1]
  Transform Pin RO : sm_lib/Frames and Transforms/Rigid Transform  TranslationMethod=None  TranslationStandardOffset=0  TranslationLengthUnit=m  TranslationStandardAxis=+Z  TranslationCartesianOffset=[0 0 0]  TranslationROffset=0  TranslationROffsetUnits=m  TranslationZOffset=0  TranslationZOffsetUnits=m  TranslationThetaOffset=0  TranslationThetaOffsetUnits=deg  RotationMethod=StandardAxis  RotationAngleUnits=deg  RotationStandardAxis=+Z  RotationAngle=180  RotationArbitraryAxis=[0 0 1]  FollAlignAxisA=+X  BaseAlignAxisA=+Y  FollAlignAxisB=+Y  BaseAlignAxisB=+Z  RotationSequenceAxes=FollowerAxes  RotationSequence=XYX  RotationSequenceAngles=[0 0 0]  RotationSequenceAnglesUnits=deg  RotationMatrix=[1 0 0; 0 1 0; 0 0 1]
  LO : PMIOPort  Side=Right
  LI : PMIOPort  Port=2  Side=Right
  RI : PMIOPort  Port=3  Side=Right
  RO : PMIOPort  Port=4  Side=Right
  H : PMIOPort  Port=5  Side=Left
  LF : PMIOPort  Port=6  Side=Left
  RF : PMIOPort  Port=7  Side=Left
  LR : PMIOPort  Port=8  Side=Left
  RR : PMIOPort  Port=9  Side=Left
  LS : Outport  VectorParamsAs1DForOutWhenUnconnected=off
  wires:
  Str/1 -> Cart/1(St)
  Dr/1 -> Cart/2(Dr)
  Limit Switch Height/1(Up) -> [LSh]
  Limit Switch Angle/1(a) -> Bus Creator/2  "LS Roll"
  [LSh] -> Bus Creator/1  "LS Height"
  Bus Creator/1 -> LS/1
  connections:
  Transform Pin RO/RConn1 -- RO/RConn1
  Cart/LConn3 -- RI/RConn1
  Pris Roller RO/LConn1 -- Cart/LConn4
  Pris Roller LO/LConn1 -- Cart/LConn1
  Pris Roller LO/RConn1 -- Roller LO/LConn1
  Pris Roller RO/RConn1 -- Roller RO/LConn1
  LO/RConn1 -- Transform Pin LO/RConn1
  LI/RConn1 -- Cart/LConn2
  Joint Limit/LConn2 -- Pris Roller RO/RConn3
  Pris Roller RO/RConn2 -- Limit Switch Height/LConn1 -- Joint Limit/LConn1
  Joint Limit/RConn1 -- Pris Roller RO/LConn2
  Limit Switch Angle/LConn1 -- Cart/RConn1 -- H/RConn1
  LF/RConn1 -- Cart/RConn3
  RF/RConn1 -- Cart/RConn4
  LR/RConn1 -- Cart/RConn2
  RR/RConn1 -- Cart/RConn5
  Roller RO/RConn1 -- Transform Pin RO/LConn1
  Transform Pin LO/LConn1 -- Roller LO/RConn1

== system sm_scissor_lift_testenv/Scissor Lift/Floor ==
  Floor : Subsystem  Tag=CustomStyle
  Initial Height : Subsystem
  Terminator{,1..3} (4 alike) : Terminator
  Wheel Floor LF : Contact_Forces_Lib/3D/Sphere to Plane Force  sphere_rad=SCL_Par.Cart.Axle.Tire.Radius/100  plane_lenx=SCL_Par.Floor.Width  plane_leny=SCL_Par.Floor.Length  plane_depth=SCL_Par.Floor.Height/2  force_law=Linear  k_contact=SCL_Par.Cart.Axle.Tire.Stiffness  b_contact=SCL_Par.Cart.Axle.Tire.Damping  pen_full_damp_F=1e-4  pen_exponent=1  custom_param_1=1  custom_param_2=1  friction_law=Stick-Slip Continuous  mu_kinetic=SCL_Par.Cart.Axle.Tire.MuKinetic  mu_static=SCL_Par.Cart.Axle.Tire.MuStatic  v_thr=SCL_Par.Cart.Axle.Tire.MuVth  vis_on=off  vis_opc_en=0  vis_len_plaBz=0.01*0.2  vis_clr=[0.9 0.2 0.2]  vis_opc=0.7
  Wheel Floor LR : Contact_Forces_Lib/3D/Sphere to Plane Force  sphere_rad=SCL_Par.Cart.Axle.Tire.Radius/100  plane_lenx=SCL_Par.Floor.Width  plane_leny=SCL_Par.Floor.Length  plane_depth=SCL_Par.Floor.Height/2  force_law=Linear  k_contact=SCL_Par.Cart.Axle.Tire.Stiffness  b_contact=SCL_Par.Cart.Axle.Tire.Damping  pen_full_damp_F=1e-4  pen_exponent=1  custom_param_1=1  custom_param_2=1  friction_law=Stick-Slip Continuous  mu_kinetic=SCL_Par.Cart.Axle.Tire.MuKinetic  mu_static=SCL_Par.Cart.Axle.Tire.MuStatic  v_thr=SCL_Par.Cart.Axle.Tire.MuVth  vis_on=off  vis_opc_en=0  vis_len_plaBz=0.01*0.2  vis_clr=[0.9 0.2 0.2]  vis_opc=0.7
  Wheel Floor RF : Contact_Forces_Lib/3D/Sphere to Plane Force  sphere_rad=SCL_Par.Cart.Axle.Tire.Radius/100  plane_lenx=SCL_Par.Floor.Width  plane_leny=SCL_Par.Floor.Length  plane_depth=SCL_Par.Floor.Height/2  force_law=Linear  k_contact=SCL_Par.Cart.Axle.Tire.Stiffness  b_contact=SCL_Par.Cart.Axle.Tire.Damping  pen_full_damp_F=1e-4  pen_exponent=1  custom_param_1=1  custom_param_2=1  friction_law=Stick-Slip Continuous  mu_kinetic=SCL_Par.Cart.Axle.Tire.MuKinetic  mu_static=SCL_Par.Cart.Axle.Tire.MuStatic  v_thr=SCL_Par.Cart.Axle.Tire.MuVth  vis_on=off  vis_opc_en=0  vis_len_plaBz=0.01*0.2  vis_clr=[0.9 0.2 0.2]  vis_opc=0.7
  Wheel Floor RR : Contact_Forces_Lib/3D/Sphere to Plane Force  sphere_rad=SCL_Par.Cart.Axle.Tire.Radius/100  plane_lenx=SCL_Par.Floor.Width  plane_leny=SCL_Par.Floor.Length  plane_depth=SCL_Par.Floor.Height/2  force_law=Linear  k_contact=SCL_Par.Cart.Axle.Tire.Stiffness  b_contact=SCL_Par.Cart.Axle.Tire.Damping  pen_full_damp_F=1e-4  pen_exponent=1  custom_param_1=1  custom_param_2=1  friction_law=Stick-Slip Continuous  mu_kinetic=SCL_Par.Cart.Axle.Tire.MuKinetic  mu_static=SCL_Par.Cart.Axle.Tire.MuStatic  v_thr=SCL_Par.Cart.Axle.Tire.MuVth  vis_on=off  vis_opc_en=0  vis_len_plaBz=0.01*0.2  vis_clr=[0.9 0.2 0.2]  vis_opc=0.7
  H : PMIOPort  Side=Left
  LR : PMIOPort  Port=2  Side=Left
  LF : PMIOPort  Port=3  Side=Left
  RF : PMIOPort  Port=4  Side=Left
  RR : PMIOPort  Port=5  Side=Left
  W : PMIOPort  Port=6  Side=Right
  wires:
  Wheel Floor LR/1 -> Terminator3/1
  Wheel Floor RR/1 -> Terminator/1
  Wheel Floor RF/1 -> Terminator1/1
  Wheel Floor LF/1 -> Terminator2/1
  connections:
  Wheel Floor RR/LConn1 -- RR/RConn1
  LR/RConn1 -- Wheel Floor LR/LConn1
  Wheel Floor LF/RConn1 -- Wheel Floor LR/RConn1 -- Initial Height/RConn1 -- Wheel Floor RF/RConn1 -- Floor/LConn1 -- Wheel Floor RR/RConn1
  Floor/RConn1 -- W/RConn1
  H/RConn1 -- Initial Height/LConn1
  Wheel Floor RF/LConn1 -- RF/RConn1
  LF/RConn1 -- Wheel Floor LF/LConn1

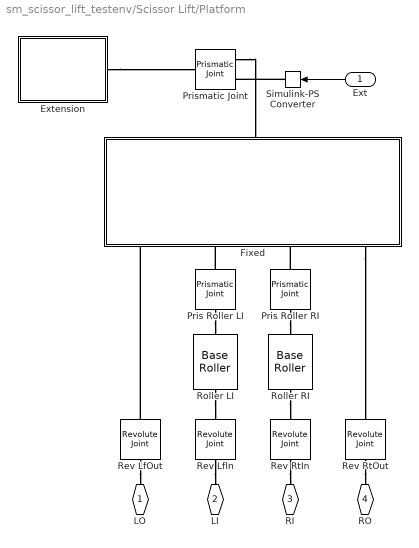
== system sm_scissor_lift_testenv/Scissor Lift/Platform ==
  Ext : Inport
  Extension : Subsystem
      mask Display: image('Scissor_Lift_Platform_Extension_IMAGE.jpg');
  Fixed : Subsystem
      mask Display: image('Scissor_Lift_Platform_Fixed_IMAGE.jpg');
  Pris Roller LI : sm_lib/Joints/Prismatic Joint  JointMode=Normal  SenseConstraintForce=off  SenseConstraintForceX=off  SenseConstraintForceY=off  SenseConstraintForceZ=off  SenseConstraintTorque=off  SenseConstraintTorqueX=off  SenseConstraintTorqueY=off  SenseConstraintTorqueZ=off  SenseTotalForce=off  SenseTotalForceX=off  SenseTotalForceY=off  SenseTotalForceZ=off  SenseTotalTorque=off  SenseTotalTorqueX=off  SenseTotalTorqueY=off  SenseTotalTorqueZ=off  CompositeWrenchDir=FollowerOnBase  CompositeWrenchFrame=BaseFrame  EquilibriumPosition=0  EquilibriumPositionUnits=m  SpringStiffness=0  SpringStiffnessUnits=N/m  DampingCoefficient=0  DampingCoefficientUnits=N/(m/s)  TorqueActuationMode=NoTorque  MotionActuationMode=ComputedMotion  SensePosition=off  SenseVelocity=off  SenseAcceleration=off  SenseTorqueForce=off  SenseLowerLimitTorqueForce=off  SenseUpperLimitTorqueForce=off  LowerLimitSpecify=off  LowerLimitBound=-1  LowerLimitBoundUnits=m  LowerLimitStiffness=1e6  LowerLimitStiffnessUnits=N/m  LowerLimitDamping=1e3  LowerLimitDampingUnits=N/(m/s)  LowerLimitTransitionRegionWidth=1e-4  LowerLimitTransitionRegionWidthUnits=m  UpperLimitSpecify=off  UpperLimitBound=1  UpperLimitBoundUnits=m  UpperLimitStiffness=1e6  UpperLimitStiffnessUnits=N/m  UpperLimitDamping=1e3  UpperLimitDampingUnits=N/(m/s)  UpperLimitTransitionRegionWidth=1e-4  UpperLimitTransitionRegionWidthUnits=m  PositionTargetSpecify=off  PositionTargetPriority=High  PositionTargetValue=-SCL_Par.Init.Roller_Position  PositionTargetValueUnits=cm  VelocityTargetSpecify=off  VelocityTargetPriority=High  VelocityTargetValue=0  VelocityTargetValueUnits=m/s
  Pris Roller RI : sm_lib/Joints/Prismatic Joint  JointMode=Normal  SenseConstraintForce=off  SenseConstraintForceX=off  SenseConstraintForceY=off  SenseConstraintForceZ=off  SenseConstraintTorque=off  SenseConstraintTorqueX=off  SenseConstraintTorqueY=off  SenseConstraintTorqueZ=off  SenseTotalForce=off  SenseTotalForceX=off  SenseTotalForceY=off  SenseTotalForceZ=off  SenseTotalTorque=off  SenseTotalTorqueX=off  SenseTotalTorqueY=off  SenseTotalTorqueZ=off  CompositeWrenchDir=FollowerOnBase  CompositeWrenchFrame=BaseFrame  EquilibriumPosition=0  EquilibriumPositionUnits=m  SpringStiffness=0  SpringStiffnessUnits=N/m  DampingCoefficient=0  DampingCoefficientUnits=N/(m/s)  TorqueActuationMode=NoTorque  MotionActuationMode=ComputedMotion  SensePosition=off  SenseVelocity=off  SenseAcceleration=off  SenseTorqueForce=off  SenseLowerLimitTorqueForce=off  SenseUpperLimitTorqueForce=off  LowerLimitSpecify=off  LowerLimitBound=-1  LowerLimitBoundUnits=m  LowerLimitStiffness=1e6  LowerLimitStiffnessUnits=N/m  LowerLimitDamping=1e3  LowerLimitDampingUnits=N/(m/s)  LowerLimitTransitionRegionWidth=1e-4  LowerLimitTransitionRegionWidthUnits=m  UpperLimitSpecify=off  UpperLimitBound=1  UpperLimitBoundUnits=m  UpperLimitStiffness=1e6  UpperLimitStiffnessUnits=N/m  UpperLimitDamping=1e3  UpperLimitDampingUnits=N/(m/s)  UpperLimitTransitionRegionWidth=1e-4  UpperLimitTransitionRegionWidthUnits=m  PositionTargetSpecify=off  PositionTargetPriority=High  PositionTargetValue=-SCL_Par.Init.Roller_Position  PositionTargetValueUnits=cm  VelocityTargetSpecify=off  VelocityTargetPriority=High  VelocityTargetValue=0  VelocityTargetValueUnits=m/s
  Prismatic Joint : sm_lib/Joints/Prismatic Joint  JointMode=Normal  SenseConstraintForce=off  SenseConstraintForceX=off  SenseConstraintForceY=off  SenseConstraintForceZ=off  SenseConstraintTorque=off  SenseConstraintTorqueX=off  SenseConstraintTorqueY=off  SenseConstraintTorqueZ=off  SenseTotalForce=off  SenseTotalForceX=off  SenseTotalForceY=off  SenseTotalForceZ=off  SenseTotalTorque=off  SenseTotalTorqueX=off  SenseTotalTorqueY=off  SenseTotalTorqueZ=off  CompositeWrenchDir=FollowerOnBase  CompositeWrenchFrame=BaseFrame  EquilibriumPosition=0  EquilibriumPositionUnits=m  SpringStiffness=0  SpringStiffnessUnits=N/m  DampingCoefficient=0  DampingCoefficientUnits=N/(m/s)  TorqueActuationMode=ComputedTorque  MotionActuationMode=InputMotion  SensePosition=off  SenseVelocity=off  SenseAcceleration=off  SenseTorqueForce=off  SenseLowerLimitTorqueForce=off  SenseUpperLimitTorqueForce=off  LowerLimitSpecify=off  LowerLimitBound=-1  LowerLimitBoundUnits=m  LowerLimitStiffness=1e6  LowerLimitStiffnessUnits=N/m  LowerLimitDamping=1e3  LowerLimitDampingUnits=N/(m/s)  LowerLimitTransitionRegionWidth=1e-4  LowerLimitTransitionRegionWidthUnits=m  UpperLimitSpecify=off  UpperLimitBound=1  UpperLimitBoundUnits=m  UpperLimitStiffness=1e6  UpperLimitStiffnessUnits=N/m  UpperLimitDamping=1e3  UpperLimitDampingUnits=N/(m/s)  UpperLimitTransitionRegionWidth=1e-4  UpperLimitTransitionRegionWidthUnits=m  PositionTargetSpecify=off  PositionTargetPriority=High  PositionTargetValue=0  PositionTargetValueUnits=m  VelocityTargetSpecify=off  VelocityTargetPriority=High  VelocityTargetValue=0  VelocityTargetValueUnits=m/s
  Rev LfIn : sm_lib/Joints/Revolute Joint  JointMode=Normal  SenseConstraintForce=off  SenseConstraintForceX=off  SenseConstraintForceY=off  SenseConstraintForceZ=off  SenseConstraintTorque=off  SenseConstraintTorqueX=off  SenseConstraintTorqueY=off  SenseConstraintTorqueZ=off  SenseTotalForce=off  SenseTotalForceX=off  SenseTotalForceY=off  SenseTotalForceZ=off  SenseTotalTorque=off  SenseTotalTorqueX=off  SenseTotalTorqueY=off  SenseTotalTorqueZ=off  CompositeWrenchDir=FollowerOnBase  CompositeWrenchFrame=BaseFrame  EquilibriumPosition=0  EquilibriumPositionUnits=rad  SpringStiffness=0  SpringStiffnessUnits=N*m/rad  DampingCoefficient=0  DampingCoefficientUnits=N*m/(rad/s)  TorqueActuationMode=NoTorque  MotionActuationMode=ComputedMotion  SensePosition=off  SenseVelocity=off  SenseAcceleration=off  SenseTorqueForce=off  SenseLowerLimitTorqueForce=off  SenseUpperLimitTorqueForce=off  LowerLimitSpecify=off  LowerLimitBound=-90  LowerLimitBoundUnits=deg  LowerLimitStiffness=1e4  LowerLimitStiffnessUnits=N*m/deg  LowerLimitDamping=10  LowerLimitDampingUnits=N*m/(deg/s)  LowerLimitTransitionRegionWidth=0.1  LowerLimitTransitionRegionWidthUnits=deg  UpperLimitSpecify=off  UpperLimitBound=90  UpperLimitBoundUnits=deg  UpperLimitStiffness=1e4  UpperLimitStiffnessUnits=N*m/deg  UpperLimitDamping=10  UpperLimitDampingUnits=N*m/(deg/s)  UpperLimitTransitionRegionWidth=0.1  UpperLimitTransitionRegionWidthUnits=deg  PositionTargetSpecify=off  PositionTargetPriority=High  PositionTargetValue=SCL_Par.Init.Base_Angle  PositionTargetValueUnits=deg  VelocityTargetSpecify=off  VelocityTargetPriority=High  VelocityTargetValue=0  VelocityTargetValueUnits=rad/s
  Rev LfOut : sm_lib/Joints/Revolute Joint  JointMode=Normal  SenseConstraintForce=off  SenseConstraintForceX=off  SenseConstraintForceY=off  SenseConstraintForceZ=off  SenseConstraintTorque=off  SenseConstraintTorqueX=off  SenseConstraintTorqueY=off  SenseConstraintTorqueZ=off  SenseTotalForce=off  SenseTotalForceX=off  SenseTotalForceY=off  SenseTotalForceZ=off  SenseTotalTorque=off  SenseTotalTorqueX=off  SenseTotalTorqueY=off  SenseTotalTorqueZ=off  CompositeWrenchDir=FollowerOnBase  CompositeWrenchFrame=BaseFrame  EquilibriumPosition=0  EquilibriumPositionUnits=rad  SpringStiffness=0  SpringStiffnessUnits=N*m/rad  DampingCoefficient=0  DampingCoefficientUnits=N*m/(rad/s)  TorqueActuationMode=NoTorque  MotionActuationMode=ComputedMotion  SensePosition=off  SenseVelocity=off  SenseAcceleration=off  SenseTorqueForce=off  SenseLowerLimitTorqueForce=off  SenseUpperLimitTorqueForce=off  LowerLimitSpecify=off  LowerLimitBound=-90  LowerLimitBoundUnits=deg  LowerLimitStiffness=1e4  LowerLimitStiffnessUnits=N*m/deg  LowerLimitDamping=10  LowerLimitDampingUnits=N*m/(deg/s)  LowerLimitTransitionRegionWidth=0.1  LowerLimitTransitionRegionWidthUnits=deg  UpperLimitSpecify=off  UpperLimitBound=90  UpperLimitBoundUnits=deg  UpperLimitStiffness=1e4  UpperLimitStiffnessUnits=N*m/deg  UpperLimitDamping=10  UpperLimitDampingUnits=N*m/(deg/s)  UpperLimitTransitionRegionWidth=0.1  UpperLimitTransitionRegionWidthUnits=deg  PositionTargetSpecify=off  PositionTargetPriority=Low  PositionTargetValue=0  PositionTargetValueUnits=deg  VelocityTargetSpecify=off  VelocityTargetPriority=High  VelocityTargetValue=0  VelocityTargetValueUnits=rad/s
  Rev RtIn : sm_lib/Joints/Revolute Joint  JointMode=Normal  SenseConstraintForce=off  SenseConstraintForceX=off  SenseConstraintForceY=off  SenseConstraintForceZ=off  SenseConstraintTorque=off  SenseConstraintTorqueX=off  SenseConstraintTorqueY=off  SenseConstraintTorqueZ=off  SenseTotalForce=off  SenseTotalForceX=off  SenseTotalForceY=off  SenseTotalForceZ=off  SenseTotalTorque=off  SenseTotalTorqueX=off  SenseTotalTorqueY=off  SenseTotalTorqueZ=off  CompositeWrenchDir=FollowerOnBase  CompositeWrenchFrame=BaseFrame  EquilibriumPosition=0  EquilibriumPositionUnits=rad  SpringStiffness=0  SpringStiffnessUnits=N*m/rad  DampingCoefficient=0  DampingCoefficientUnits=N*m/(rad/s)  TorqueActuationMode=NoTorque  MotionActuationMode=ComputedMotion  SensePosition=off  SenseVelocity=off  SenseAcceleration=off  SenseTorqueForce=off  SenseLowerLimitTorqueForce=off  SenseUpperLimitTorqueForce=off  LowerLimitSpecify=off  LowerLimitBound=-90  LowerLimitBoundUnits=deg  LowerLimitStiffness=1e4  LowerLimitStiffnessUnits=N*m/deg  LowerLimitDamping=10  LowerLimitDampingUnits=N*m/(deg/s)  LowerLimitTransitionRegionWidth=0.1  LowerLimitTransitionRegionWidthUnits=deg  UpperLimitSpecify=off  UpperLimitBound=90  UpperLimitBoundUnits=deg  UpperLimitStiffness=1e4  UpperLimitStiffnessUnits=N*m/deg  UpperLimitDamping=10  UpperLimitDampingUnits=N*m/(deg/s)  UpperLimitTransitionRegionWidth=0.1  UpperLimitTransitionRegionWidthUnits=deg  PositionTargetSpecify=off  PositionTargetPriority=Low  PositionTargetValue=0  PositionTargetValueUnits=deg  VelocityTargetSpecify=off  VelocityTargetPriority=High  VelocityTargetValue=0  VelocityTargetValueUnits=rad/s
  Rev RtOut : sm_lib/Joints/Revolute Joint  JointMode=Normal  SenseConstraintForce=off  SenseConstraintForceX=off  SenseConstraintForceY=off  SenseConstraintForceZ=off  SenseConstraintTorque=off  SenseConstraintTorqueX=off  SenseConstraintTorqueY=off  SenseConstraintTorqueZ=off  SenseTotalForce=off  SenseTotalForceX=off  SenseTotalForceY=off  SenseTotalForceZ=off  SenseTotalTorque=off  SenseTotalTorqueX=off  SenseTotalTorqueY=off  SenseTotalTorqueZ=off  CompositeWrenchDir=FollowerOnBase  CompositeWrenchFrame=BaseFrame  EquilibriumPosition=0  EquilibriumPositionUnits=rad  SpringStiffness=0  SpringStiffnessUnits=N*m/rad  DampingCoefficient=0  DampingCoefficientUnits=N*m/(rad/s)  TorqueActuationMode=NoTorque  MotionActuationMode=ComputedMotion  SensePosition=off  SenseVelocity=off  SenseAcceleration=off  SenseTorqueForce=off  SenseLowerLimitTorqueForce=off  SenseUpperLimitTorqueForce=off  LowerLimitSpecify=off  LowerLimitBound=-90  LowerLimitBoundUnits=deg  LowerLimitStiffness=1e4  LowerLimitStiffnessUnits=N*m/deg  LowerLimitDamping=10  LowerLimitDampingUnits=N*m/(deg/s)  LowerLimitTransitionRegionWidth=0.1  LowerLimitTransitionRegionWidthUnits=deg  UpperLimitSpecify=off  UpperLimitBound=90  UpperLimitBoundUnits=deg  UpperLimitStiffness=1e4  UpperLimitStiffnessUnits=N*m/deg  UpperLimitDamping=10  UpperLimitDampingUnits=N*m/(deg/s)  UpperLimitTransitionRegionWidth=0.1  UpperLimitTransitionRegionWidthUnits=deg  PositionTargetSpecify=off  PositionTargetPriority=Low  PositionTargetValue=-SCL_Par.Init.Base_Angle  PositionTargetValueUnits=deg  VelocityTargetSpecify=off  VelocityTargetPriority=High  VelocityTargetValue=0  VelocityTargetValueUnits=rad/s
  Roller LI : sm_scissor_lift_lib/Base Roller  roller_length=SCL_Par.Roller.Roller_Length  roller_radius=SCL_Par.Roller.Roller_Radius  shaft_length=SCL_Par.Roller.Shaft_Length  shaft_radius=SCL_Par.Roller.Shaft_Radius  material_density=SCL_Par.Roller.Density  material_color=SCL_Par.Roller.Color  material_opacity=SCL_Par.Roller.Opacity
      settings: SourceProductName=Simscape Scissor Lift Library
  Roller RI : sm_scissor_lift_lib/Base Roller  roller_length=SCL_Par.Roller.Roller_Length  roller_radius=SCL_Par.Roller.Roller_Radius  shaft_length=SCL_Par.Roller.Shaft_Length  shaft_radius=SCL_Par.Roller.Shaft_Radius  material_density=SCL_Par.Roller.Density  material_color=SCL_Par.Roller.Color  material_opacity=SCL_Par.Roller.Opacity
      settings: SourceProductName=Simscape Scissor Lift Library
  Simulink-PS Converter : nesl_utility/Simulink-PS Converter  PhysicalDomain=network_engine_domain  SubClassName=ps_input  LeftPortType=input  RightPortType=output  PseudoPeriodic=off  Frequencies=[]  NoiseDistribution=none  NoiseParameters=[]  Unit=m  AffineConversion=off  FilteringAndDerivatives=filter  SimscapeFilterOrder=2  InputFilterTimeConstant=0.005  UdotUserProvided=0
      settings: SourceProductBaseCode=PW,SS
  LO : PMIOPort  Side=Left
  LI : PMIOPort  Port=2  Side=Left
  RI : PMIOPort  Port=3  Side=Left
  RO : PMIOPort  Port=4  Side=Left
  wires:
  Ext/1 -> Simulink-PS Converter/1
  connections:
  Rev RtOut/LConn1 -- RO/RConn1
  Rev LfIn/LConn1 -- LI/RConn1
  Rev LfOut/LConn1 -- LO/RConn1
  Rev RtIn/LConn1 -- RI/RConn1
  Rev LfOut/RConn1 -- Fixed/LConn1
  Fixed/LConn4 -- Rev RtOut/RConn1
  Extension/RConn1 -- Prismatic Joint/RConn1
  Prismatic Joint/LConn1 -- Fixed/RConn1
  Simulink-PS Converter/RConn1 -- Prismatic Joint/LConn2
  Pris Roller RI/RConn1 -- Roller RI/LConn1
  Roller RI/RConn1 -- Rev RtIn/RConn1
  Roller LI/RConn1 -- Rev LfIn/RConn1
  Pris Roller LI/RConn1 -- Roller LI/LConn1
  Pris Roller RI/LConn1 -- Fixed/LConn3
  Pris Roller LI/LConn1 -- Fixed/LConn2
